simulink model "msd_07_Simscape_2"  (R2026a)
settings: Solver=VariableStepAuto  MaxStep=0.01  AbsTol=1e-3
InitFcn:
  | m = 3.600;  % kg
  | k = 400;    % N/m
  | b = 10;     % Ns/m
libraries: fl_lib x7, nesl_utility x3
Description:
  | Copyright 2017-2026 The MathWorks, Inc.
settings Model: Creator=smiller  LastModifiedBy=smiller
settings ConfigComp: CovMetricSettings=dswe
settings SimscapeCC: SimscapeNormalizeSystem=off  SimscapeNominalValues="[{\"value\":\"1\",\"unit\":\"A\"},{\"value\":\"1\",\"unit\":\"bar\"},{\"value\":\"1\",\"unit\":\"cm^2\"},{\"value\":\"1\",\"unit\":\"cm^3/s\"},{\"value\":\"1\",\"unit\":\"kJ/kg\"},{\"value\":\"1\",\"unit\":\"kW\"},{\"value\":\"1\",\"unit\":\"l\"},{\"value\":\"1\",\"unit\":\"N\"},{\"value\":\"1\",\"unit\":\"N*m\"},{\"value\":\"1\",\"unit\":\"V\"}]"

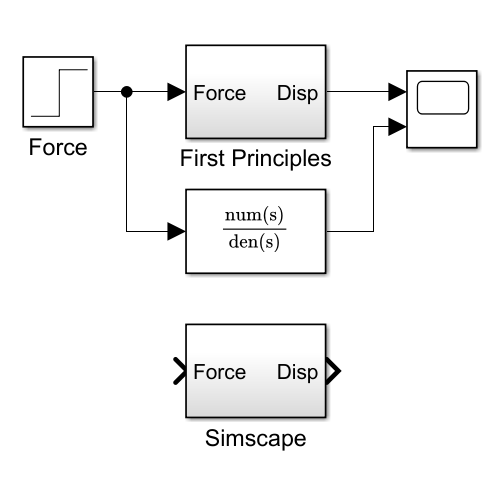
[thumbnail: Simulink's stored preview of the top-level diagram]
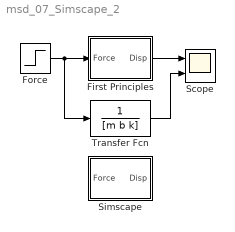
== system msd_07_Simscape_2 ==
  First Principles : Subsystem
  Force : Step  FinalValue=10  SampleTime=0
  Scope : Scope  NumInputPorts=2
      settings: ActiveDisplayYMinimum=-0.00518  ActiveDisplayYMaximum=0.04665
  Simscape : Subsystem
  Transfer Fcn : TransferFcn  Denominator=[m b k]
  wires:
  Force/1 -> Transfer Fcn/1, First Principles/1(Force)
  First Principles/1(Disp) -> Scope/1
  Transfer Fcn/1 -> Scope/2

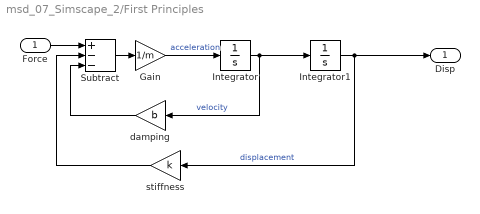
== system msd_07_Simscape_2/First Principles ==
  Force : Inport
  Gain : Gain  Gain=1/m
  Integrator : Integrator
  Integrator1 : Integrator
  Subtract : Sum  Inputs=+--
  damping : Gain  Gain=b
  stiffness : Gain  Gain=k
  Disp : Outport  VectorParamsAs1DForOutWhenUnconnected=off
  wires:
  damping/1 -> Subtract/3
  Force/1 -> Subtract/1
  Subtract/1 -> Gain/1
  Gain/1 -> Integrator/1  "acceleration"
  Integrator/1 -> damping/1, Integrator1/1  "velocity"
  stiffness/1 -> Subtract/2
  Integrator1/1 -> Disp/1, stiffness/1  "displacement"

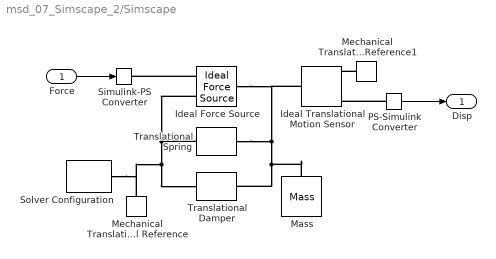
== system msd_07_Simscape_2/Simscape ==
  Force : Inport
  Ideal Force Source : fl_lib/Mechanical/Mechanical Sources/Ideal Force Source
  Ideal Translational Motion Sensor : fl_lib/Mechanical/Mechanical Sensors/Ideal Translational Motion Sensor  reference=foundation.enum.MeasurementReference.difference  acceleration_port=false  velocity_port=true  position_port=true  offset=0 m
  Mass : fl_lib/Mechanical/Translational Elements/Mass  mass=m kg  num_ports=foundation.enum.numPorts2.one  v_specify=off  v_priority=High  v=0 m/s  v_nominal_specify=off  v_nominal_value=1  v_nominal_unit=m/s  f_specify=off  f_priority=None  f=0 N  f_nominal_specify=off  f_nominal_value=1  f_nominal_unit=N
  Mechanical Translational Reference : fl_lib/Mechanical/Translational Elements/Mechanical Translational Reference
  Mechanical Translational Reference1 : fl_lib/Mechanical/Translational Elements/Mechanical Translational Reference
  PS-Simulink Converter : nesl_utility/PS-Simulink Converter  PhysicalDomain=network_engine_domain  SubClassName=ps_output  LeftPortType=input  RightPortType=output  PseudoPeriodic=off  Frequencies=[]  VectorFormat=1-D array  Unit=m  AffineConversion=off
  Simulink-PS Converter : nesl_utility/Simulink-PS Converter  PhysicalDomain=network_engine_domain  SubClassName=ps_input  LeftPortType=input  RightPortType=output  PseudoPeriodic=off  Frequencies=[]  NoiseDistribution=none  NoiseParameters=[]  Unit=N  AffineConversion=off  FilteringAndDerivatives=zero  SimscapeFilterOrder=1  InputFilterTimeConstant=0.001  UdotUserProvided=1
  Solver Configuration : nesl_utility/Solver Configuration  PhysicalDomain=network_engine_domain  SubClassName=solver  LeftPortType=input  RightPortType=generic  Tones=[]  Harmonics=[]  SimulateNoise=off  Profile=off  UseLocalSampling=off  EnableSwitchedLinearOptims=on  FrequencyDomain=off  UseCCode=off  RelTol=0.001  AbsTol=1e-06  MinStep=1e-09  ToWorkspace=off  RevertToSquareIcSolve=off  NumHomotopyIterations=100  PhasorMode=off  PhasorModeNumHarmonics=1  ConsistencySolver=NEWTON_FTOL  CanonicalOrdering=UNORDERED  OptimizeIntermediates=UNOPTIMIZED  IndexReductionMethod=DerivativeReplacement  DoDC=off  ResidualTolerance=1e-09  ConsistencyTolSource=GLOBAL  ConsistencyAbsTol=0.001  ConsistencyRelTol=0.001  ConsistencyTolFactor=0.001  UseLocalSolver=off  LocalSolverChoice=NE_BACKWARD_EULER_ADVANCER  ResolveIndetEquations=on  FunctionEvalNumThread=1  LocalSolverSampleTime=0.001  DoFixedCost=off  MaxNonlinIter=3  MaxModeIter=2  ComputeImpulses=off  ImpulseIterations=2  LinearAlgebra=Sparse  LinearAlgebraNumThread=0  EquationFormulation=NE_TIME_EF  DelaysMemoryBudget=1024  AutomaticFiltering=on  FilteringTimeConstant=0.001  PartitionStorageMethod=AS_NEEDED  PartitionMemoryBudget=1024  PartitionMethod=FAST  MultibodyUseLocalSolver=off  MultibodyLocalSolverChoice=ODE1  MultibodyLocalSolverSampleTime=0.001
  Translational Damper : fl_lib/Mechanical/Translational Elements/Translational Damper  D=b N/(m/s)  v_specify=off  v_priority=None  v=0 m/s  v_nominal_specify=off  v_nominal_value=1  v_nominal_unit=m/s  f_specify=off  f_priority=None  f=0 N  f_nominal_specify=off  f_nominal_value=1  f_nominal_unit=N
  Translational Spring : fl_lib/Mechanical/Translational Elements/Translational Spring  spr_rate=k N/m  v_specify=off  v_priority=None  v=0 m/s  v_nominal_specify=off  v_nominal_value=1  v_nominal_unit=m/s  f_specify=off  f_priority=None  f=0 N  f_nominal_specify=off  f_nominal_value=1  f_nominal_unit=N  x_specify=off  x_priority=High  x=0 m  x_nominal_specify=off  x_nominal_value=1  x_nominal_unit=m
  Disp : Outport  VectorParamsAs1DForOutWhenUnconnected=off
  wires:
  Force/1 -> Simulink-PS Converter/1
  PS-Simulink Converter/1 -> Disp/1
  connections:
  Translational Spring/LConn1 -- Ideal Force Source/RConn2 -- Mechanical Translational Reference/LConn1 -- Solver Configuration/RConn1 -- Translational Damper/LConn1
  Translational Spring/RConn1 -- Ideal Translational Motion Sensor/LConn1 -- Ideal Force Source/LConn1 -- Mass/LConn1 -- Translational Damper/RConn1
  Ideal Force Source/RConn1 -- Simulink-PS Converter/RConn1
  Mechanical Translational Reference1/LConn1 -- Ideal Translational Motion Sensor/RConn1
  PS-Simulink Converter/LConn1 -- Ideal Translational Motion Sensor/RConn3
